simulink model "Coba_Lagi"  (R2022b)
settings: Solver=VariableStepAuto  StartTime=0.0  StopTime=3600  RelTol=1e-3
undefined symbols (not defined in the file): Ion, Lithium
libraries: spsBatteryLib x1, spsCurrentMeasurementLib x1, spsDCVoltageSourceLib x1, spsGroundLib x1, spsVoltageMeasurementLib x1, sps_lib x1
settings Model: Creator=Haposan  LastModifiedBy=Haposan

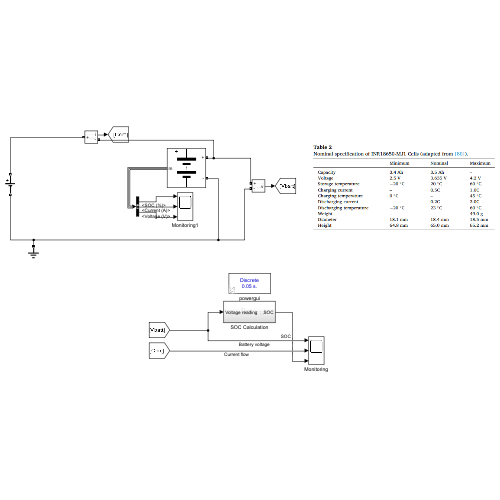
[thumbnail: Simulink's stored preview of the top-level diagram]
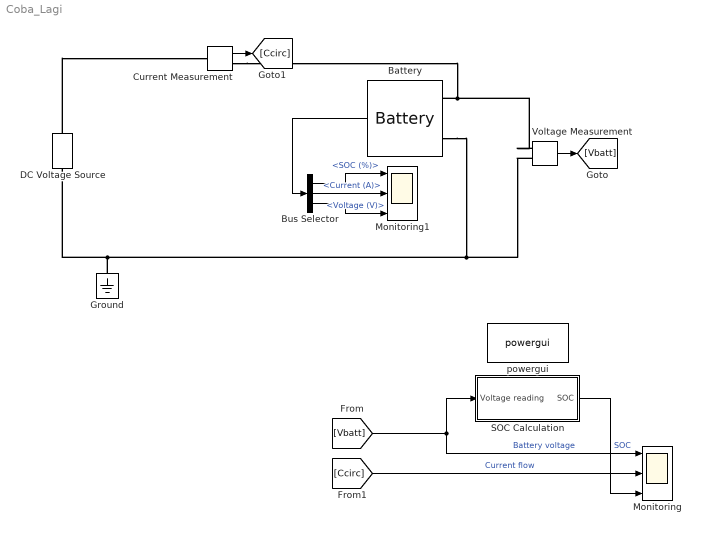
== system Coba_Lagi ==
  Battery : spsBatteryLib/Battery  BatType=Lithium-Ion  ShowTempParam=off  ThermalPreset=no  ShowAgeParam=off  NomV=3.635  NomQ=3.5  SOC=10  Batt_Tr=1  PresetModel=on  MaxQ=3.5  MinV=2.7262  FullV=4.2311  Dis_rate=1.5217  R=0.010386  Normal_OP=3.1652  expZone="[3.9272     0.17196]"  current=[6.5 13 32.5]  Units=Time  Tci=20  NomT=20  T2=-30  MaxQ2=4.8  FullV2=7.1  Normal_OP2=5.655  expZone2="[6.58           1]"  Rca=0.6  ti=2000  Dp=0  Neq0=0  Tsim=1e6  Ta1=25  Qeol=5.4*0.9  Reol=0.013333*1.2  Char_age=[2.3478, 3]  Dis_age=[2.3478, 10]  N1=1500  N2=10500  N3=1000  N4=1400  Ta2=45  N5=950
  Bus Selector : BusSelector  OutputSignals=SOC (%),Current (A),Voltage (V)
  Current Measurement : spsCurrentMeasurementLib/Current Measurement  PhasorSimulation=off  OutputType=Complex  PSBequivalent=0
  DC Voltage Source : spsDCVoltageSourceLib/DC Voltage Source  Amplitude=5  Measurements=None
  Ground : spsGroundLib/Ground  LConnTagsString=a
  Monitoring : Scope  NumInputPorts=3
  Monitoring1 : Scope  NumInputPorts=3
  SOC Calculation : Subsystem
  Voltage Measurement : spsVoltageMeasurementLib/Voltage Measurement  PhasorSimulation=off  OutputType=Complex  PSBequivalent=0
  powergui : sps_lib/powergui  Priority=1  SimulationMode=Discrete  SampleTime=50e-3  frequency=60  Iterations=50  frequencyindice=0  Pbase=100e6  ErrMax=1e-4  UnitsV=kV  UnitsW=MW  buscounter=0  FunctionMessages=off  echomessages=off  EnableUseOfTLC=off  CurrentSourceSwitches=off  DisableSnubberDevices=off  DisableRonSwitches=off  DisableVfSwitches=off  DisplayEquations=off  AutomaticDiscreteSolvers=off  SolverType=Tustin/Backward Euler (TBE)  Interpol=off  ExternalGateDelay=off  methode=off  Ts=100  x0status=blocks  SPID=on  SwTol=0  HookPort=off  NonlinearTolerance=1e-4  nMaxIteration=100  ContinueOnMaxIteration=off  RestoreLinks=warning  ResistiveCurrentMeasurement=off  Frange=[0:2:500]  Ylog=off  Xlog=on  ShowGrid=off  save=off  variable=ZData  structure=0  ZoomFFT=off  StartTime=0.0  cycles=1  DisplayStyle=1  fundamental=60  FreqAxis=off  MaxFrequency=1000  frequencyindicesteady=1  RmsSteady=1  display=off
  wires:
  [Ccirc] -> Monitoring/2  "Current flow"
  [Vbatt] -> SOC Calculation/1(Voltage reading), Monitoring/1  "Battery voltage"
  SOC Calculation/1(SOC) -> Monitoring/3  "SOC"
  Voltage Measurement/1 -> [Vbatt]
  Current Measurement/1 -> [Ccirc]
  Battery/1 -> Bus Selector/1
  Bus Selector/1 -> Monitoring1/1  "<SOC (%)>"
  Bus Selector/2 -> Monitoring1/2  "<Current (A)>"
  Bus Selector/3 -> Monitoring1/3  "<Voltage (V)>"
  connections:
  DC Voltage Source/RConn1 -- Current Measurement/LConn1
  Current Measurement/RConn1 -- Voltage Measurement/LConn1 -- Battery/LConn1
  Battery/LConn2 -- Voltage Measurement/LConn2 -- Ground/LConn1 -- DC Voltage Source/LConn1

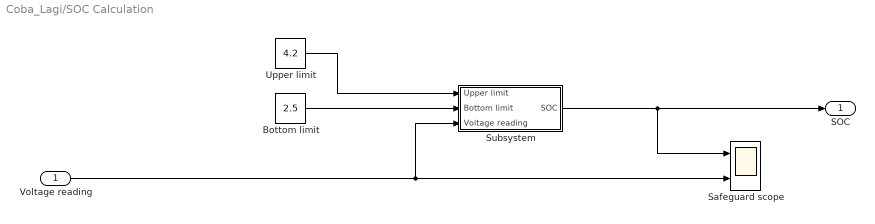
== system Coba_Lagi/SOC Calculation ==
  Voltage reading : Inport
  Bottom limit : Constant  Value=2.5
  Safeguard scope : Scope  NumInputPorts=2
  Subsystem : Subsystem
  Upper limit : Constant  Value=4.2
  SOC : Outport
  wires:
  Bottom limit/1 -> Subsystem/2(Bottom limit)
  Voltage reading/1 -> Safeguard scope/2, Subsystem/3(Voltage reading)
  Upper limit/1 -> Subsystem/1(Upper limit)
  Subsystem/1(SOC) -> Safeguard scope/1, SOC/1

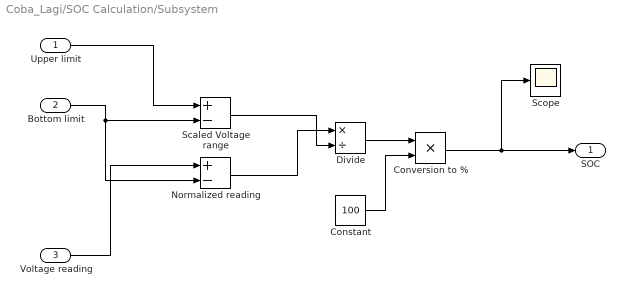
== system Coba_Lagi/SOC Calculation/Subsystem ==
  Upper limit : Inport
  Bottom limit : Inport  Port=2
  Voltage reading : Inport  Port=3
  Constant : Constant  Value=100
  Conversion to % : Product
  Divide : Product  Inputs=*/
  Normalized reading : Sum  Inputs=+-
  Scaled Voltage range : Sum  Inputs=+-
  Scope : Scope
  SOC : Outport
  wires:
  Upper limit/1 -> Scaled Voltage range/1
  Bottom limit/1 -> Normalized reading/2, Scaled Voltage range/2
  Voltage reading/1 -> Normalized reading/1
  Normalized reading/1 -> Divide/1
  Scaled Voltage range/1 -> Divide/2
  Divide/1 -> Conversion to %/1
  Constant/1 -> Conversion to %/2
  Conversion to %/1 -> Scope/1, SOC/1
